simulink model "InnerOuter_Sim"  (Simulink 6.6)
settings: Solver=ode4  StartTime=0.0  StopTime=125  FixedStep=SampleT  RelTol=1e-3
InitFcn:
  | clc
  | innerOuterInit
undefined symbols (not defined in the file): A1, Apolar, apSampleTime, bankCommandLimit, baseHeight, baseTemp, CD0, chord, CL0, CLa, CLa_dot, Clb, ClDa, CLDe, CLDf, ClDr, clock, Clp, CLq, Clr, Cm0, Cma, CmDe, CmDf, Cmq, Cnb, CnDa, CnDr, Cnp, Cnr, compensatorOn, CYb, CYDr, da_failamp, da_failbias, da_failper, daL_fail, daLimit, daR_fail, deg, deLimit, derivativesConstant, dr_fail, dr_failamp, dr_failbias, dr_failper, drLimit, dtLimit, Earth, elarm, Euler_0, F, gaind, getWP, ISA_g, Ixx, Iyy, Izz, L1OF, L2_base ... (+28)
libraries: simulink x102, SLUGS_Library x23, aerolibconvert2 x15, dsPICdrivers x8, aerolibactuator x5, aerolibtransform2 x2, aerolibwind2 x2, dspmtrx3 x2, aerolibatmos2 x1, aerolibutil x1
(part 1 of 4)
CloseFcn:
  | rtwprivate ssgencode ModelCloseRequest AttitudeComplementary
settings Model: Creator=ASL_Lab  LastModifiedBy=Administrator
settings DebuggingCC: ConsistencyChecking=warning  AlgebraicLoopMsg=error  MultiTaskDSMMsg=warning  MultiTaskCondExecSysMsg=none  ModelReferenceExtraNoncontSigs=warning  StrictBusMsg=None
settings HardwareCC: TargetHWDeviceType=32-bit Generic
settings RTWCC: IncludeERTFirstTime=on

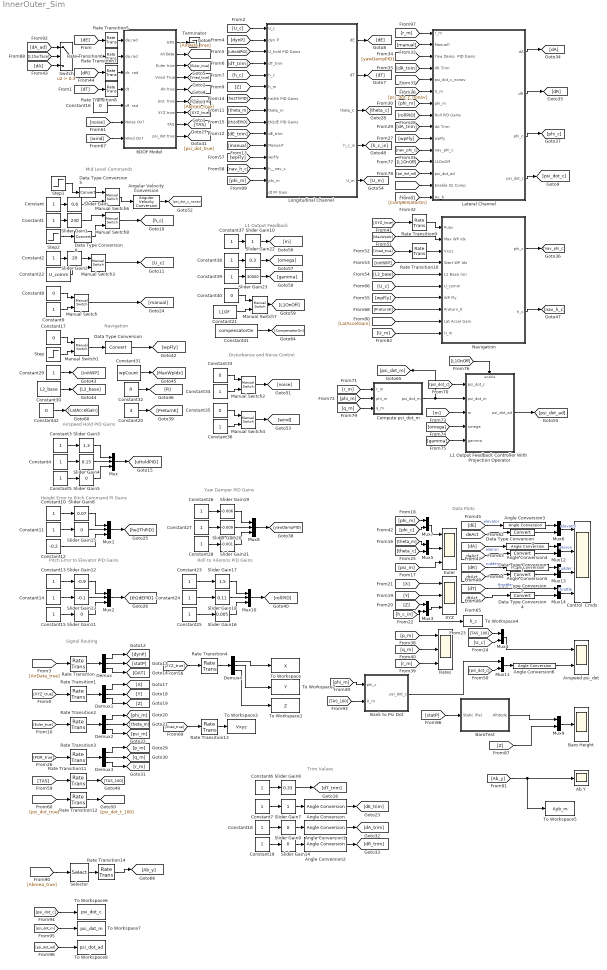
== system InnerOuter_Sim ==
  note: Mid Level Commands
  note: Trim Values
  note: Signal Routing
  note: Airspeed Hold PID Gains
  note: Height Error to Pitch Command PI Gains
  note: Pitch Error to Elevator PID Gains
  note: Data Plots
  note: Yaw Damper PID Gains
  note: Roll to Ailerons PID Gains
  note: Navigation
  note: Disturbance and Noise Control
  note: L1 Output Feedback
  6DOF Model : Subsystem
  Ab Y : Scope
      settings: TimeRange=140  YMin=-3  YMax=3  SaveName=ScopeData9
  Airspeed psi_dot : Scope  NumInputPorts=2
      settings: TimeRange=125  YMin=14.91~-37.5  YMax=15.05~5  SaveName=AirspeedPsiDot
  Angle Conversion : aerolibconvert2/Angle Conversion  SystemSampleTime=-1  IU=deg  OU=rad
  Angle Conversion1 : aerolibconvert2/Angle Conversion  SystemSampleTime=-1  IU=deg  OU=rad
  Angle Conversion2 : aerolibconvert2/Angle Conversion  SystemSampleTime=-1  IU=deg  OU=rad
  Angle Conversion{3..6} (4 alike) : aerolibconvert2/Angle Conversion  SystemSampleTime=-1  IU=rad  OU=deg
  Angular Velocity Conversion : aerolibconvert2/Angular Velocity Conversion  SystemSampleTime=-1  IU=deg/s  OU=rad/s
  Bank to Psi Dot : Subsystem  AncestorBlock=SLUGS_Library/Navigation/Bank to Psi Dot
  Baro Height : Scope
      settings: TimeRange=350  YMin=-1500  YMax=700  SaveName=AirspeedPsiDot1
  BaroTest : Subsystem
  Compute psi_dot_m : Subsystem
  Constant{,1..7,10..11,13..15,18..19,23..28,37..39} (24 alike) : Constant  OutDataTypeMode=single  SampleTime=apSampleTime
  Constant12 : Constant  Value=-0.2  OutDataTypeMode=single  SampleTime=apSampleTime
  Constant16 : Constant  Value=0
  Constant17 : Constant  Value=0  OutDataTypeMode=uint8  SampleTime=apSampleTime
  Constant20 : Constant  Value=4  SampleTime=apSampleTime
  Constant21 : Constant  Value=L1OF  SampleTime=apSampleTime
  Constant22 : Constant  Value=U_comm  SampleTime=apSampleTime
  Constant29 : Constant  OutDataTypeMode=uint8  SampleTime=apSampleTime
  Constant30 : Constant  Value=L2_base  OutDataTypeMode=single  SampleTime=apSampleTime
  Constant31 : Constant  Value=wpCount  SampleTime=apSampleTime
  Constant32 : Constant  Value=R  SampleTime=apSampleTime
  Constant33 : Constant  Value=0  SampleTime=SampleT
  Constant34 : Constant  SampleTime=SampleT
  Constant35 : Constant  Value=0  SampleTime=SampleT
  Constant36 : Constant  SampleTime=SampleT
  Constant40 : Constant  Value=0  OutDataTypeMode=uint8  SampleTime=apSampleTime
  Constant41 : Constant  Value=compensatorOn  SampleTime=apSampleTime
  Constant42 : Constant  Value=0  SampleTime=apSampleTime
  Constant8 : Constant  Value=0  OutDataTypeMode=uint8  SampleTime=apSampleTime
  Constant9 : Constant  OutDataTypeMode=uint8  SampleTime=apSampleTime
  Control  Cmds : Scope  NumInputPorts=4
      settings: TickLabels=on  TimeRange=100  YMin=-2~-10~-11~0.225  YMax=3.5~17.5~1~0.425  SaveName=ctrlCmds
  Data Type Conversion : DataTypeConversion  OutDataTypeMode=uint8
  Data Type Conversion{1..6} (6 alike) : DataTypeConversion  OutDataTypeMode=single
  Demux{,1..4} (5 alike) : Demux  Outputs=3
  Euler : Scope  NumInputPorts=3
      settings: TimeRange=100  YMin=-0.4~-0.02~0  YMax=1~0.06~7  SaveName=EulerData  DataFormat=Structure
  L1 Output Feedback Controller With  Projection Operator : Subsystem  TreatAsAtomicUnit=on
  Lateral Channel : Subsystem  TreatAsAtomicUnit=on
  Longitudinal Channel : Subsystem  TreatAsAtomicUnit=on
  Manual Switch{,2,4,6..8} (6 alike) : simulink/Signal Routing/Manual Switch  SystemSampleTime=-1  sw=1  action=0  varsize=off
  Manual Switch1 : simulink/Signal Routing/Manual Switch  SystemSampleTime=-1  sw=0  action=0  varsize=off
  Manual Switch3 : simulink/Signal Routing/Manual Switch  SystemSampleTime=-1  sw=0  action=0  varsize=off
  Mux{,1..2,8,10} (5 alike) : Mux  Inputs=3
  Mux{3..7,9,11..14} (10 alike) : Mux  Inputs=2
  Navigation : Subsystem  TreatAsAtomicUnit=on
  Rate Transition{,1..4,9..14} (11 alike) : RateTransition  OutPortSampleTime=apSampleTime
  Rate Transition{5..8} (4 alike) : RateTransition  OutPortSampleTime=SampleT
  Rates : Scope  NumInputPorts=3
      settings: TimeRange=300  YMin=-0.75~-1.5~-0.3  YMax=1~1.5~0.7  SaveName=ScopeData3
  Selector : Selector  IndexOptions=Index vector (dialog)  Indices=[2]  OutputSizes=1  InputPortWidth=3
  Slider Gain : simulink/Math Operations/Slider Gain  SystemSampleTime=-1  low=-18  gain=0.6  high=18
  Slider Gain1 : simulink/Math Operations/Slider Gain  SystemSampleTime=-1  low=0  gain=230  high=800
  Slider Gain10 : simulink/Math Operations/Slider Gain  SystemSampleTime=-1  low=0  gain=1  high=10
  Slider Gain11 : simulink/Math Operations/Slider Gain  SystemSampleTime=-1  low=-0.1  gain=0  high=0
  Slider Gain12 : simulink/Math Operations/Slider Gain  SystemSampleTime=-1  low=-2  gain=-0.9  high=0.3
  Slider Gain13 : simulink/Math Operations/Slider Gain  SystemSampleTime=-1  low=-0.1  gain=-0.1  high=0
  Slider Gain14 : simulink/Math Operations/Slider Gain  SystemSampleTime=-1  low=-10  gain=0  high=10
  Slider Gain15 : simulink/Math Operations/Slider Gain  SystemSampleTime=-1  low=-20  gain=0  high=20
  Slider Gain16 : simulink/Math Operations/Slider Gain  SystemSampleTime=-1  low=-0.1  gain=0.005  high=0.1
  Slider Gain17 : simulink/Math Operations/Slider Gain  SystemSampleTime=-1  low=-0.1  gain=1.5  high=5
  Slider Gain18 : simulink/Math Operations/Slider Gain  SystemSampleTime=-1  low=0  gain=0.11  high=2
  Slider Gain19 : simulink/Math Operations/Slider Gain  SystemSampleTime=-1  low=-20  gain=-0.006  high=20
  Slider Gain2 : simulink/Math Operations/Slider Gain  SystemSampleTime=-1  low=1  gain=20  high=55
  Slider Gain20 : simulink/Math Operations/Slider Gain  SystemSampleTime=-1  low=-20  gain=-0.009  high=20
  Slider Gain21 : simulink/Math Operations/Slider Gain  SystemSampleTime=-1  low=-20  gain=-0.001  high=20
  Slider Gain22 : simulink/Math Operations/Slider Gain  SystemSampleTime=-1  low=0  gain=0.3  high=5
  Slider Gain23 : simulink/Math Operations/Slider Gain  SystemSampleTime=-1  low=-50000  gain=30000  high=50000
  Slider Gain3 : simulink/Math Operations/Slider Gain  SystemSampleTime=-1  low=0  gain=1.3  high=4.5
  Slider Gain4 : simulink/Math Operations/Slider Gain  SystemSampleTime=-1  low=-20  gain=0.15  high=20
  Slider Gain5 : simulink/Math Operations/Slider Gain  SystemSampleTime=-1  low=-20  gain=0  high=20
  Slider Gain6 : simulink/Math Operations/Slider Gain  SystemSampleTime=-1  low=0.1  gain=0.33  high=1
  Slider Gain7 : simulink/Math Operations/Slider Gain  SystemSampleTime=-1  low=-10  gain=1  high=10
  Slider Gain8 : simulink/Math Operations/Slider Gain  SystemSampleTime=-1  low=-20  gain=0.07  high=20
  Slider Gain9 : simulink/Math Operations/Slider Gain  SystemSampleTime=-1  low=-10  gain=0  high=10
  Step : Step  Time=2  SampleTime=0.01
  Step1 : Step  Time=10  After=5  SampleTime=0.01
  Step2 : Step  Time=10  Before=Pos_0(3)  After=500  SampleTime=0.01
  Switch : Switch  Criteria=u2 > Threshold  Threshold=0.3  SampleTime=apSampleTime  InputSameDT=on
  Terminator : Terminator
  To Workspace : ToWorkspace  VariableName=X  SampleTime=-1  SaveFormat=Array
  To Workspace1 : ToWorkspace  VariableName=Z  SampleTime=-1  SaveFormat=Array
  To Workspace2 : ToWorkspace  VariableName=Y  SampleTime=-1  SaveFormat=Array
  To Workspace3 : ToWorkspace  VariableName=Vxyz  SampleTime=-1  SaveFormat=Array
  To Workspace4 : ToWorkspace  VariableName=h_c  SampleTime=-1  SaveFormat=Array
  To Workspace5 : ToWorkspace  VariableName=Ayb_m  SampleTime=.01  SaveFormat=Array
  To Workspace6 : ToWorkspace  VariableName=psi_dot_c  SampleTime=.01  SaveFormat=Array
  To Workspace7 : ToWorkspace  VariableName=psi_dot_m  SampleTime=.01  SaveFormat=Array
  To Workspace8 : ToWorkspace  VariableName=psi_dot_ad  SampleTime=.01  SaveFormat=Array
  XYZ : Scope  NumInputPorts=3
      settings: TimeRange=125  YMin=-250~-200~180  YMax=100~200~230
  wires:
  6DOF Model/7(XYZ true) -> [XYZ_true]
  6DOF Model/4(Vned True) -> [Vned_true]
  6DOF Model/5(Ab true) -> [Abmea_true]
  6DOF Model/6("pqr, true") -> [PQR_true]
  6DOF Model/3(Euler true) -> [Euler_true]
  6DOF Model/2(AirData) -> [AirData_true]
  Longitudinal Channel/1(dE) -> [dE]
  Longitudinal Channel/2(dT) -> [dT]
  Constant/1 -> Slider Gain/1
  Constant1/1 -> Slider Gain1/1
  Constant2/1 -> Slider Gain2/1
  Angular Velocity Conversion/1 -> [psi_dot_c_nonav]
  [U_c] -> Longitudinal Channel/1(U_c)
  [AirData_true] -> Rate Transition/1
  Demux/1 -> [dynP]
  Demux/2 -> [statP]
  Demux/3 -> [OAT]
  Constant3/1 -> Slider Gain3/1
  Constant4/1 -> Slider Gain4/1
  Constant5/1 -> Slider Gain5/1
  Slider Gain4/1 -> Mux/2
  Slider Gain3/1 -> Mux/1
  Slider Gain5/1 -> Mux/3
  Mux/1 -> [uHoldPID]
  [dynP] -> Longitudinal Channel/2(dyn P)
  [uHoldPID] -> Longitudinal Channel/3(U_hold PID Gains)
  Constant6/1 -> Slider Gain6/1
  Slider Gain6/1 -> [dT_trim]
  [dT_trim] -> Longitudinal Channel/4(dT_trim)
  [h_c] -> Longitudinal Channel/5(h_c)
  [XYZ_true] -> Rate Transition1/1
  Demux1/1 -> [X]
  Demux1/2 -> [Y]
  Demux1/3 -> [Z]
  [Z] -> Longitudinal Channel/6(h_m)
  [Euler_true] -> Rate Transition2/1
  Demux2/1 -> [phi_m]
  Demux2/2 -> [theta_m]
  Demux2/3 -> [psi_m]
  [theta_m] -> Longitudinal Channel/8(theta_m)
  Constant7/1 -> Slider Gain7/1
  Slider Gain7/1 -> Angle Conversion/1
  Angle Conversion/1 -> [dE_trim]
  [dE_trim] -> Longitudinal Channel/10(dE_trim)
  Constant8/1 -> Manual Switch/1
  Constant9/1 -> Manual Switch/2
  Manual Switch/1 -> [manual]
  [manual] -> Longitudinal Channel/11(Manual?)
  Constant10/1 -> Slider Gain8/1
  Constant11/1 -> Slider Gain15/1
  Constant12/1 -> Mux1/3
  Slider Gain8/1 -> Mux1/1
  Mux1/1 -> [he2ThPID]
  Constant13/1 -> Slider Gain12/1
  Constant14/1 -> Slider Gain13/1
  Constant15/1 -> Slider Gain11/1
  Slider Gain13/1 -> Mux2/2
  Slider Gain12/1 -> Mux2/1
  Slider Gain11/1 -> Mux2/3
  Mux2/1 -> [th2dEPID]
  [he2ThPID] -> Longitudinal Channel/7(he2th PID Gains)
  [th2dEPID] -> Longitudinal Channel/9(th2dE PID Gains)
  Mux5/1 -> Euler/2
  [psi_m] -> Euler/3
  [X] -> XYZ/1
  [Y] -> XYZ/2
  Mux3/1 -> XYZ/3
  [Z] -> Mux3/1
  [h_c_in] -> Mux3/2, To Workspace4/1
  [dT] -> Rate Transition8/1
  [dE] -> Rate Transition5/1
  Mux4/1 -> Airspeed psi_dot/1
  6DOF Model/8(TAS) -> [TAS]
  [TAS_100] -> Mux4/1
  [U_c] -> Mux4/2
  [theta_c] -> Mux5/2
  Longitudinal Channel/3(theta_C) -> [theta_c]
  [PQR_true] -> Rate Transition3/1
  Demux3/1 -> [p_m]
  Demux3/2 -> [q_m]
  Demux3/3 -> [r_m]
  Constant18/1 -> Slider Gain9/1
  Slider Gain9/1 -> Angle Conversion1/1
  Angle Conversion1/1 -> [dA_trim]
  Constant19/1 -> Slider Gain14/1
  Slider Gain14/1 -> Angle Conversion2/1
  Angle Conversion2/1 -> [dR_trim]
  [Ab_y] -> Lateral Channel/15(Ay_b)
  [manual] -> Lateral Channel/2(Manual?)
  [yawDampPID] -> Lateral Channel/3(Yaw Damp  PID Gains)
  [dR_trim] -> Lateral Channel/4(dR Trim)
  [psi_dot_c_nonav] -> Lateral Channel/5(psi_dot_c_nonav)
  [U_m] -> Lateral Channel/6(U_m)
  [phi_m] -> Lateral Channel/7(phi_m)
  [rollPID] -> Lateral Channel/8(Roll PID Gains)
  [dA_trim] -> Lateral Channel/9(dA Trim)
  [r_m] -> Rates/3
  Lateral Channel/3(phi_c) -> [phi_c]
  [q_m] -> Rates/2
  [phi_m] -> Mux7/1
  [phi_c] -> Mux7/2
  Mux7/1 -> Euler/1
  Constant26/1 -> Slider Gain19/1
  Constant27/1 -> Slider Gain20/1
  Constant28/1 -> Slider Gain21/1
  Slider Gain20/1 -> Mux8/2
  Slider Gain19/1 -> Mux8/1
  Slider Gain21/1 -> Mux8/3
  Mux8/1 -> [yawDampPID]
  Constant23/1 -> Slider Gain17/1
  Constant24/1 -> Slider Gain18/1
  Constant25/1 -> Slider Gain16/1
  Slider Gain18/1 -> Mux10/2
  Slider Gain17/1 -> Mux10/1
  Slider Gain16/1 -> Mux10/3
  Mux10/1 -> [rollPID]
  Switch/1 -> Rate Transition6/1
  [dR] -> Rate Transition7/1
  Constant16/1 -> 6DOF Model/5("df, rad")
  Slider Gain15/1 -> Mux1/2
  Mux6/1 -> Control  Cmds/1  "elevator"
  Mux12/1 -> Control  Cmds/2  "aileron"
  [theta_m] -> Mux5/1
  6DOF Model/9(psi_dot true) -> [psi_dot_true]
  Bank to Psi Dot/1(psi_dot_c) -> Mux11/1
  [psi_dot_c] -> Mux11/2
  Mux11/1 -> Angle Conversion6/1
  [p_m] -> Rates/1
  Constant17/1 -> Manual Switch1/1
  Step/1 -> Manual Switch1/2
  Manual Switch1/1 -> Data Type Conversion/1
  Constant29/1 -> [initWP]
  [wpFly] -> Lateral Channel/10(wpFly)
  Navigation/1(phi_c) -> [nav_phi_c]
  [nav_phi_c] -> Lateral Channel/11(nav_phi_c)
  [XYZ_true] -> Rate Transition9/1
  Constant30/1 -> [L2_base]
  Constant31/1 -> [MaxWpIdx]
  [Vned_true] -> Rate Transition10/1
  [L2_base] -> Navigation/5(L2 Base (m))
  [XYZ_true] -> Rate Transition4/1
  Demux4/1 -> To Workspace/1
  Demux4/2 -> To Workspace2/1
  Demux4/3 -> To Workspace1/1
  Navigation/2(h_c) -> [nav_h_c]
  [wpFly] -> Longitudinal Channel/12(wpFly)
  [nav_h_c] -> Longitudinal Channel/13(h__nav_c)
  Longitudinal Channel/4(h_c_in) -> [h_c_in]
  Rate Transition/1 -> Demux/1
  Rate Transition1/1 -> Demux1/1
  Rate Transition2/1 -> Demux2/1
  Rate Transition3/1 -> Demux3/1
  Rate Transition4/1 -> Demux4/1
  Rate Transition9/1 -> Navigation/1(Puav)
  Rate Transition10/1 -> Navigation/3(Vxyz)
  [TAS] -> Rate Transition11/1
  Rate Transition11/1 -> [TAS_100]
  [psi_dot_true] -> Rate Transition12/1
  Rate Transition12/1 -> [psi_dot_t_100]
  Constant33/1 -> Manual Switch2/1
  Constant34/1 -> Manual Switch2/2
  Manual Switch2/1 -> [noise]
  [noise] -> 6DOF Model/6(Noise On?)
  Constant32/1 -> [R]
  [U_c] -> Navigation/6(U_comm)
  6DOF Model/1(GPS) -> Terminator/1
  [wpFly] -> Navigation/7(WP Fly)
  Slider Gain2/1 -> Manual Switch3/1
  Manual Switch3/1 -> [U_c]
  Constant22/1 -> Manual Switch3/2
  [dE] -> Angle Conversion3/1  "elevator"
  [deAct] -> Data Type Conversion3/1
  [dA] -> Angle Conversion4/1  "aileron"
  [daAct] -> Data Type Conversion1/1
  Mux13/1 -> Control  Cmds/3  "rudder"
  [dR] -> Angle Conversion5/1  "rudder"
  [drAct] -> Data Type Conversion2/1
  Mux14/1 -> Control  Cmds/4  "throttle"
  [dT] -> Mux14/1  "throttle"
  [dtAct] -> Data Type Conversion4/1
  Lateral Channel/4("psi_dot_c ") -> [psi_dot_c]
  Constant35/1 -> Manual Switch4/1
  Constant36/1 -> Manual Switch4/2
  Manual Switch4/1 -> [wind]
  [wind] -> 6DOF Model/7(Wind On?)
  Longitudinal Channel/5(U_m) -> [U_m]
  Data Type Conversion/1 -> [wpFly]
  Lateral Channel/1(dA) -> [dA]
  Lateral Channel/2(dR) -> [dR]
  Data Type Conversion3/1 -> Mux6/2
  Data Type Conversion1/1 -> Mux12/2
  Data Type Conversion2/1 -> Mux13/2
  Data Type Conversion4/1 -> Mux14/2
  Rate Transition5/1 -> 6DOF Model/1(de,rad)
  Rate Transition8/1 -> 6DOF Model/4(dt)
  Rate Transition6/1 -> 6DOF Model/2(da,rad)
  Rate Transition7/1 -> 6DOF Model/3("dr, rad")
  Rate Transition13/1 -> To Workspace3/1
  [Vned_true] -> Rate Transition13/1
  Manual Switch6/1 -> Angular Velocity Conversion/1
  Slider Gain/1 -> Manual Switch6/2
  Step1/1 -> Data Type Conversion5/1
  Data Type Conversion5/1 -> Manual Switch6/1
  [psi_dot_c] -> L1 Output Feedback Controller With  Projection Operator/1(psi_dot_c)
  L1 Output Feedback Controller With  Projection Operator/1(psi_dot_ad) -> [psi_dot_ad]
  [phi_m] -> Compute psi_dot_m/2(phi_m)
  [r_m] -> Compute psi_dot_m/1(r_m)
  Constant37/1 -> Slider Gain10/1
  Slider Gain10/1 -> [m]
  Constant38/1 -> Slider Gain22/1
  Slider Gain22/1 -> [omega]
  Constant39/1 -> Slider Gain23/1
  Slider Gain23/1 -> [gamma]
  [m] -> L1 Output Feedback Controller With  Projection Operator/3(m)
  [omega] -> L1 Output Feedback Controller With  Projection Operator/4(omega)
  [gamma] -> L1 Output Feedback Controller With  Projection Operator/5(gamma)
  Constant40/1 -> Manual Switch7/1
  Constant21/1 -> Manual Switch7/2
  Manual Switch7/1 -> [L1OnOff]
  [L1OnOff] -> Lateral Channel/12(L1OnOff)
  [psi_dot_ad] -> Lateral Channel/13(psi_dot_ad)
  [L1OnOff] -> L1 Output Feedback Controller With  Projection Operator/Enable
  [q_m] -> Compute psi_dot_m/3(q_m)
  Compute psi_dot_m/1(psi_dot_m) -> L1 Output Feedback Controller With  Projection Operator/2(psi_dot_m), [psi_dot_m]
  Angle Conversion3/1 -> Mux6/1
  Angle Conversion4/1 -> Mux12/1
  Angle Conversion5/1 -> Mux13/1
  [dA] -> Switch/3
  [dA_ad] -> Switch/1
  [L1Surface] -> Switch/2
  Constant41/1 -> [CompensatorOn]
  [CompensatorOn] -> Lateral Channel/14(Enable SS Comp)
  Manual Switch8/1 -> [h_c]
  Step2/1 -> Data Type Conversion6/1
  Slider Gain1/1 -> Manual Switch8/1
  Data Type Conversion6/1 -> Manual Switch8/2
  [statP] -> BaroTest/1(Static (Pa))
  Mux9/1 -> Baro Height/1
  [Z] -> Mux9/2
  BaroTest/1(Altitude) -> Mux9/1
  [phi_m] -> Longitudinal Channel/14(phi_m)
  Selector/1 -> Rate Transition14/1
  [Abmea_true] -> Selector/1
  Rate Transition14/1 -> [Ab_y]
  [Ab_y] -> Ab Y/1, To Workspace5/1
  Angle Conversion6/1 -> Airspeed psi_dot/2
  [phi_m] -> Bank to Psi Dot/1(phi_c)
  [TAS_100] -> Bank to Psi Dot/2(U_m)
  [psi_dot_c] -> To Workspace6/1
  [psi_dot_m] -> To Workspace7/1
  [psi_dot_ad] -> To Workspace8/1
  [r_m] -> Lateral Channel/1(r_m)
  [MaxWpIdx] -> Navigation/2(Max WP Idx)
  [initWP] -> Navigation/4(Start WP Idx)
  [PreturnK] -> Navigation/8(Preturn_K)
  Constant20/1 -> [PreturnK]
  Constant42/1 -> [LatAccelGain]
  [LatAccelGain] -> Navigation/9(Lat Accel Gain)
  [U_m] -> Navigation/10(U_m)

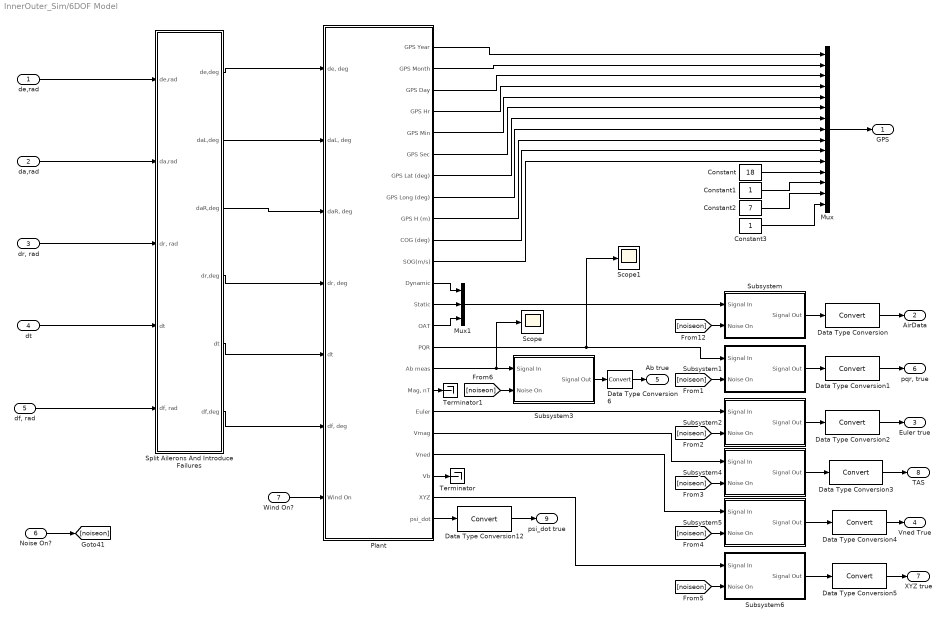
== system InnerOuter_Sim/6DOF Model ==
  de,rad : Inport
  da,rad : Inport  Port=2
  "dr, rad" : Inport  Port=3
  dt : Inport  Port=4
  "df, rad" : Inport  Port=5
  Noise On? : Inport  Port=6
  Wind On? : Inport  Port=7
  Constant : Constant  Value=18  SampleTime=SampleT
  Constant1 : Constant  SampleTime=SampleT
  Constant2 : Constant  Value=7  SampleTime=SampleT
  Constant3 : Constant  SampleTime=SampleT
  Data Type Conversion{,1..6,12} (8 alike) : DataTypeConversion  OutDataTypeMode=single
  Mux : Mux  Inputs=15
  Mux1 : Mux  Inputs=3
  Plant : Subsystem
  Scope : Scope
      settings: YMin=-13  YMax=1  SaveName=ScopeData5
  Scope1 : Scope
      settings: YMin=-0.05  YMax=0.04  SaveName=ScopeData6
  Split Ailerons And Introduce Failures : Subsystem
  Subsystem : Subsystem  mask{nv=[0.01 0.01 0.1], st=SampleT, ns=[132 564 987]}
      mask prompts: nv "Noise Variance"; st "Sample Time"; ns "Noise Seed"
  Subsystem1 : Subsystem  mask{nv=[0.001 0.001 0.001], st=SampleT, ns=[132 564 987]}
      mask prompts: nv "Noise Variance"; st "Sample Time"; ns "Noise Seed"
  Subsystem2 : Subsystem  mask{nv=[0.0001 0.00003 0.0001], st=SampleT, ns=[132 564 987]}
      mask prompts: nv "Noise Variance"; st "Sample Time"; ns "Noise Seed"
  Subsystem3 : Subsystem  mask{nv=[0.1 0.1 0.1], st=SampleT, ns=[132 564 987]}
      mask prompts: nv "Noise Variance"; st "Sample Time"; ns "Noise Seed"
  Subsystem4 : Subsystem  mask{nv=[0.01], st=SampleT, ns=[321564]}
      mask prompts: nv "Noise Variance"; st "Sample Time"; ns "Noise Seed"
  Subsystem5 : Subsystem  mask{nv=[0.01 0.01 0.01], st=SampleT, ns=[321564 6546 98798]}
      mask prompts: nv "Noise Variance"; st "Sample Time"; ns "Noise Seed"
  Subsystem6 : Subsystem  mask{nv=[0.05 0.05 0.07], st=SampleT, ns=[321564]}
      mask prompts: nv "Noise Variance"; st "Sample Time"; ns "Noise Seed"
  Terminator : Terminator
  Terminator1 : Terminator
  GPS : Outport
  AirData : Outport  Port=2
  Euler true : Outport  Port=3
  Vned True : Outport  Port=4
  Ab true : Outport  Port=5
  "pqr, true" : Outport  Port=6
  XYZ true : Outport  Port=7
  TAS : Outport  Port=8
  psi_dot true : Outport  Port=9
  wires:
  Mux/1 -> GPS/1
  Plant/1(GPS Year) -> Mux/1
  Plant/2(GPS Month) -> Mux/2
  Plant/3(GPS Day) -> Mux/3
  Plant/4(GPS Hr) -> Mux/4
  Plant/5(GPS Min) -> Mux/5
  Plant/6(GPS Sec) -> Mux/6
  Plant/7(GPS Lat (deg)) -> Mux/7
  Plant/8(GPS Long (deg)) -> Mux/8
  Plant/9(GPS H (m)) -> Mux/9
  Plant/10(COG (deg)) -> Mux/10
  Plant/11(SOG(m/s)) -> Mux/11
  Plant/12(Dynamic) -> Mux1/1
  Plant/13(Static) -> Mux1/2
  Plant/14(OAT) -> Mux1/3
  Mux1/1 -> Subsystem/1(Signal In)
  Constant/1 -> Mux/12
  Constant1/1 -> Mux/13
  Constant2/1 -> Mux/14
  Constant3/1 -> Mux/15
  Plant/23(psi_dot) -> Data Type Conversion12/1
  Noise On?/1 -> [noiseon]
  Subsystem/1(Signal Out) -> Data Type Conversion/1
  [noiseon] -> Subsystem/2(Noise On)
  [noiseon] -> Subsystem1/2(Noise On)
  [noiseon] -> Subsystem2/2(Noise On)
  [noiseon] -> Subsystem4/2(Noise On)
  [noiseon] -> Subsystem5/2(Noise On)
  [noiseon] -> Subsystem6/2(Noise On)
  [noiseon] -> Subsystem3/2(Noise On)
  Subsystem1/1(Signal Out) -> Data Type Conversion1/1
  Plant/15(PQR) -> Subsystem1/1(Signal In), Scope1/1
  Subsystem2/1(Signal Out) -> Data Type Conversion2/1
  Plant/18(Euler) -> Subsystem2/1(Signal In)
  Subsystem3/1(Signal Out) -> Data Type Conversion6/1
  Plant/16(Ab meas) -> Subsystem3/1(Signal In), Scope/1
  Subsystem4/1(Signal Out) -> Data Type Conversion3/1
  Plant/19(Vmag) -> Subsystem4/1(Signal In)
  Subsystem5/1(Signal Out) -> Data Type Conversion4/1
  Plant/20(Vned) -> Subsystem5/1(Signal In)
  Subsystem6/1(Signal Out) -> Data Type Conversion5/1
  Plant/22(XYZ) -> Subsystem6/1(Signal In)
  Plant/21(Vb) -> Terminator/1
  Plant/17("Mag, nT") -> Terminator1/1
  Split Ailerons And Introduce Failures/1(de,deg) -> Plant/1("de, deg")
  Split Ailerons And Introduce Failures/6(df,deg) -> Plant/6("df, deg")
  Split Ailerons And Introduce Failures/4(dr,deg) -> Plant/4("dr, deg")
  Split Ailerons And Introduce Failures/2(daL,deg) -> Plant/2("daL, deg")
  Wind On?/1 -> Plant/7(Wind On)
  Data Type Conversion/1 -> AirData/1
  Data Type Conversion1/1 -> "pqr, true"/1
  Data Type Conversion2/1 -> Euler true/1
  Data Type Conversion3/1 -> TAS/1
  Data Type Conversion4/1 -> Vned True/1
  Data Type Conversion5/1 -> XYZ true/1
  Data Type Conversion6/1 -> Ab true/1
  Data Type Conversion12/1 -> psi_dot true/1
  de,rad/1 -> Split Ailerons And Introduce Failures/1(de,rad)
  da,rad/1 -> Split Ailerons And Introduce Failures/2(da,rad)
  "dr, rad"/1 -> Split Ailerons And Introduce Failures/3("dr, rad")
  dt/1 -> Split Ailerons And Introduce Failures/4(dt)
  Split Ailerons And Introduce Failures/5("dt ") -> Plant/5(dt)
  "df, rad"/1 -> Split Ailerons And Introduce Failures/5("df, rad")
  Split Ailerons And Introduce Failures/3(daR,deg) -> Plant/3("daR, deg")

== system InnerOuter_Sim/Bank to Psi Dot ==
  phi_c : Inport
  U_m : Inport  Port=2
  Constant1 : Constant  Value=9.80665  OutDataTypeMode=single
  Divide : Product  Inputs=/*  OutDataTypeMode=single  OutScaling=2^-10  SampleTime=apSampleTime
  Divide1 : Product  OutDataTypeMode=single  OutScaling=2^-10  SampleTime=apSampleTime
  Subsystem8 : SLUGS_Library/Subsystem8  SystemSampleTime=-1
  negprotect : Stateflow chart
  psi_dot_c : Outport
  wires:
  negprotect/1(zpVal) -> Divide/1
  Divide/1 -> Divide1/2
  phi_c/1 -> Subsystem8/1
  Subsystem8/1 -> Divide1/1
  Divide1/1 -> psi_dot_c/1
  Constant1/1 -> Divide/2
  U_m/1 -> negprotect/1(val)

== system InnerOuter_Sim/BaroTest ==
  Static (Pa) : Inport  Orientation=up
  Compute Barometric Height : Subsystem  mask{baseTemp=baseTemp, LapseRate=lapseRate}
      mask prompts: baseTemp "Base Station Temperature (K)"; LapseRate "Lapse Rate (C/ft)"
      mask help:
      | Produces Altitude in meters from Barometric Pressure in Pascals. Altitude is valid from MSL to 6000 ft.
      |
      | The method implemented here was developed by Ren Curry
  Constant1 : Constant  Value=baseHeight  OutDataTypeMode=single
  Enables/Disables the Computation of  initial Baro Bias : Stateflow chart
  Initial Baro Bias : Subsystem  TreatAsAtomicUnit=on
  Sum1 : Sum  Inputs=++|  OutDataTypeMode=single
  Zero Out Height : Subsystem  TreatAsAtomicUnit=on
  Altitude : Outport
  wires:
  Compute Barometric Height/1("Altitude, m") -> Zero Out Height/2(Computed Height), Sum1/2
  Static (Pa)/1 -> Initial Baro Bias/1(Baro (Pa)), Compute Barometric Height/3(Baro (Pa))
  Enables/Disables the Computation of  initial Baro Bias/1(tOut) -> Initial Baro Bias/Enable, Zero Out Height/Enable
  Constant1/1 -> Compute Barometric Height/1(Base Height (m)), Zero Out Height/1(Base Height)
  Initial Baro Bias/1(Baro (Gnd)) -> Compute Barometric Height/2(Base Pressure (Pa))
  Zero Out Height/1(Height Offset) -> Sum1/1
  Sum1/1 -> Altitude/1

== system InnerOuter_Sim/Compute psi_dot_m ==
  r_m : Inport
  phi_m : Inport  Port=2
  q_m : Inport  Port=3
  Product : Product  SampleTime=apSampleTime  RndMeth=Zero
  Product1 : Product  SampleTime=apSampleTime  RndMeth=Zero
  Subsystem5 : Subsystem  AncestorBlock=SLUGS_Library/Subsystem5
  Subsystem7 : SLUGS_Library/Subsystem7  SystemSampleTime=-1
  Subtract : Sum  Inputs=2  OutScaling=2^-10
  psi_dot_m : Outport
  wires:
  Subsystem5/1(cos(u)) -> Product/2
  Subsystem7/1 -> Product1/2
  Product/1 -> Subtract/1
  Product1/1 -> Subtract/2
  r_m/1 -> Product/1
  phi_m/1 -> Subsystem5/1(u), Subsystem7/1
  Subtract/1 -> psi_dot_m/1
  q_m/1 -> Product1/1

== system InnerOuter_Sim/L1 Output Feedback Controller With  Projection Operator ==
  psi_dot_c : Inport
  psi_dot_m : Inport  Port=2
  m : Inport  Port=3
  omega : Inport  Port=4
  gamma : Inport  Port=5
  Enable : EnablePort  ShowOutputPort=on
  Constant : Constant  Value=2  OutDataTypeMode=single
  Constant1 : Constant  OutDataTypeMode=single
  Control  Law : Subsystem
      mask Display:
      | droots([],'-a','a')
      | port_label('input',1,'a')
      | port_label('input',2,'u')
      | port_label('output',1,'y')
  Gain : Gain  Gain=-1
  Integer Delay : simulink/Discrete/Integer Delay  vinit=0.0  samptime=apSampleTime  NumDelays=1
  Integer Delay1 : simulink/Discrete/Integer Delay  Orientation=left  vinit=0.0  samptime=-1  NumDelays=1
  Logical Operator : Logic  Operator=NOT  AllPortsSameDT=off  OutDataTypeMode=Specify via dialog
  Projection : Product  SampleTime=apSampleTime  RndMeth=Zero
  Projection Operator : Subsystem
  Psi Dot  Limit : Saturate  UpperLimit=1  LowerLimit=-1  SampleTime=apSampleTime
  State Predictor : Subsystem
      mask Display:
      | droots([],'-a','a')
      | port_label('input',1,'a')
      | port_label('input',2,'u')
      | port_label('output',1,'y')
  Sum2 : Sum  Inputs=|++  SampleTime=apSampleTime
  Sum3 : Sum  Inputs=-+|  SampleTime=apSampleTime
  Sum4 : Sum  Inputs=+-|  SampleTime=apSampleTime
  Trapezoidal Integrator : Subsystem  AncestorBlock=SLUGS_Library/Control Blocks/PID Controller w//Anti-Windup/Trapezoidal Integrator  mask{T=apSampleTime, upperLimit=2, lowerLimit=-2}
      mask prompts: T "Sample Time"; upperLimit "Upper Saturation"; lowerLimit "Lower Saturation"
  psi_dot_ad : Outport
  wires:
  Integer Delay1/1 -> Projection Operator/3(Theta), Sum2/2
  Constant1/1 -> Projection Operator/2(Eps 0)
  Constant/1 -> Projection Operator/1(Theta Max)
  Projection Operator/1("Proj(the, y)") -> Projection/2  "G*Proj"
  Sum4/1 -> Psi Dot  Limit/1  "psi_ad"
  Control  Law/1(y) -> Sum4/2  "sigma_hat_fil"
  omega/1 -> Control  Law/1(a)
  psi_dot_c/1 -> Integer Delay/1  "psi_dot_c"
  Trapezoidal Integrator/1(Int(x)) -> Control  Law/2(u), Integer Delay1/1  "sigma_hat"
  Projection/1 -> Trapezoidal Integrator/1(x)
  gamma/1 -> Projection/1  "adaptation gain"
  Sum3/1 -> Gain/1  "psi_dot_tilde"
  psi_dot_m/1 -> Sum3/1  "psi_dot_m"
  Sum2/1 -> State Predictor/2(u)
  m/1 -> State Predictor/1(a)
  Gain/1 -> Projection Operator/4(y)
  State Predictor/1(y) -> Sum3/2
  Integer Delay/1 -> Sum4/1  "psi_dot_c"
  Psi Dot  Limit/1 -> psi_dot_ad/1, Sum2/1
  Logical Operator/1 -> Trapezoidal Integrator/2(Reset)
  Enable/1 -> Logical Operator/1

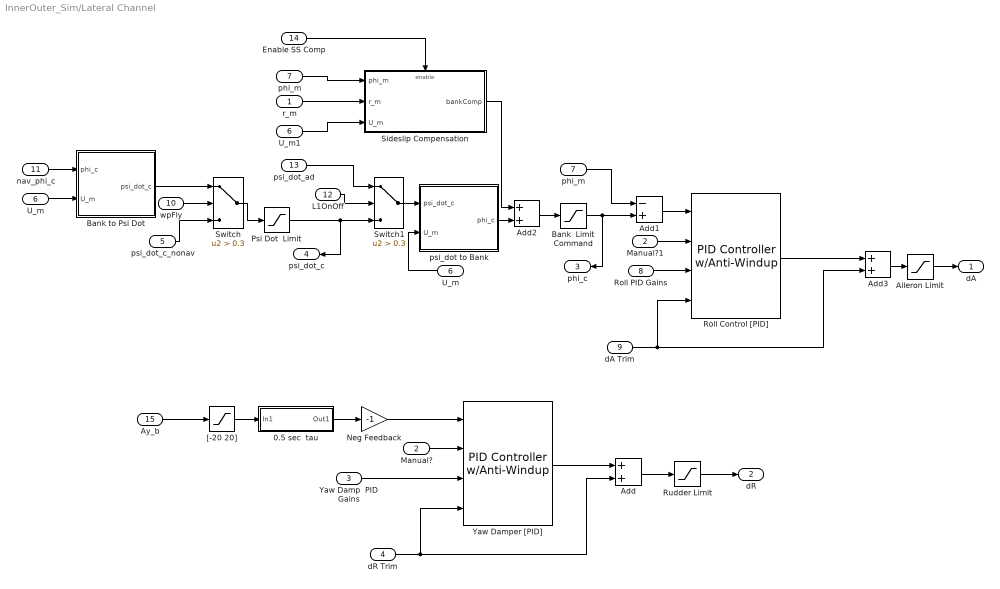
== system InnerOuter_Sim/Lateral Channel ==
  r_m : Inport
  Manual? : Inport  Port=2
  Yaw Damp  PID Gains : Inport  Port=3
  dR Trim : Inport  Port=4
  psi_dot_c_nonav : Inport  Port=5
  U_m : Inport  Port=6
  phi_m : Inport  Port=7
  Roll PID Gains : Inport  Port=8
  dA Trim : Inport  Port=9
  wpFly : Inport  Port=10  SampleTime=apSampleTime
  nav_phi_c : Inport  Port=11
  L1OnOff : Inport  Port=12  SampleTime=apSampleTime
  psi_dot_ad : Inport  Port=13  SampleTime=apSampleTime
  Enable SS Comp : Inport  Port=14
  Ay_b : Inport  Port=15
  0.5 sec  tau : Subsystem  mask(Tustin1stOrderLowpassAutoInitialCondition){f=0.3183, T=T}
      mask prompts: f "Lowpass Frequency"; T "Sample Time"
      mask help: Takes a 3db rolloff frequency (in Hz, NOT radians/s) and a sample time. Performs a symbolic Tustin conversion and implements in a discrete filter. The initial output of the filter is set by the first sample.
      mask Help: Enter the desired 3db rolloff frequency in Hz and the sample time. Initial conditions are sampled automatically.
      mask Display: fprintf('%.2f Hz lowpass',f)
  Add : Sum  OutDataTypeMode=single  OutScaling=2^-10
  Add1 : Sum  Inputs=-+  OutDataTypeMode=single  OutScaling=2^-10
  Add2 : Sum  OutDataTypeMode=single  OutScaling=2^-10
  Add3 : Sum  OutDataTypeMode=single  OutScaling=2^-10
  Aileron Limit : Saturate  UpperLimit=daLimit  LowerLimit=-daLimit  SampleTime=apSampleTime
  Bank  Limit Command : Saturate  UpperLimit=bankCommandLimit  LowerLimit=-bankCommandLimit  SampleTime=apSampleTime
  Bank to Psi Dot : Subsystem  AncestorBlock=SLUGS_Library/Navigation/Bank to Psi Dot
  Manual?1 : InportShadow  Port=2  LatchByCopyingInsideSignal=off
  Neg Feedback : Gain  Gain=-1  OutDataTypeMode=Specify via dialog  OutDataType=float('double')
  Psi Dot  Limit : Saturate  UpperLimit=1  LowerLimit=-1  SampleTime=apSampleTime
  Roll Control [PID] : SLUGS_Library/Control Blocks/PID Controller w//Anti-Windup  SystemSampleTime=-1  Tsample=apSampleTime  Ndelay=derivativesConstant  upperSaturationLimit=daLimit  lowerSaturationLimit=-daLimit
  Rudder Limit : Saturate  UpperLimit=drLimit  LowerLimit=-drLimit  SampleTime=apSampleTime
  Sideslip Compensation : Subsystem
  Switch : Switch  Criteria=u2 > Threshold  Threshold=0.3  SampleTime=apSampleTime
  Switch1 : Switch  Criteria=u2 > Threshold  Threshold=0.3  SampleTime=apSampleTime
  "U_m " : InportShadow  Orientation=left  Port=6  LatchByCopyingInsideSignal=off
  U_m1 : InportShadow  Port=6  LatchByCopyingInsideSignal=off
  Yaw Damper [PID] : SLUGS_Library/Control Blocks/PID Controller w//Anti-Windup  SystemSampleTime=-1  Tsample=apSampleTime  Ndelay=derivativesConstant  upperSaturationLimit=drLimit  lowerSaturationLimit=-drLimit
  "[-20 20]" : Saturate  UpperLimit=20  LowerLimit=-20
  "phi_m " : InportShadow  Port=7  LatchByCopyingInsideSignal=off
  psi_dot to Bank : Subsystem  AncestorBlock=SLUGS_Library/Navigation/psi_dot to Bank
  dA : Outport
  dR : Outport  Port=2
  phi_c : Outport  Orientation=left  Port=3
  "psi_dot_c " : Outport  Orientation=left  Port=4
  wires:
  Rudder Limit/1 -> dR/1
  Manual?/1 -> Yaw Damper [PID]/2
  Yaw Damp  PID Gains/1 -> Yaw Damper [PID]/3
  Add/1 -> Rudder Limit/1
  Yaw Damper [PID]/1 -> Add/1
  U_m/1 -> Bank to Psi Dot/2(U_m)
  Manual?1/1 -> Roll Control [PID]/2
  Roll PID Gains/1 -> Roll Control [PID]/3
  Add3/1 -> Aileron Limit/1
  Roll Control [PID]/1 -> Add3/1
  Aileron Limit/1 -> dA/1
  Add1/1 -> Roll Control [PID]/1
  phi_m/1 -> Add1/1
  Bank to Psi Dot/1(psi_dot_c) -> Switch/1
  wpFly/1 -> Switch/2
  Bank  Limit Command/1 -> Add1/2, phi_c/1
  nav_phi_c/1 -> Bank to Psi Dot/1(phi_c)
  Switch/1 -> Psi Dot  Limit/1
  "U_m "/1 -> psi_dot to Bank/2(U_m)
  psi_dot_c_nonav/1 -> Switch/3
  Switch1/1 -> psi_dot to Bank/1(psi_dot_c)
  L1OnOff/1 -> Switch1/2
  psi_dot_ad/1 -> Switch1/1
  "phi_m "/1 -> Sideslip Compensation/1(phi_m)
  r_m/1 -> Sideslip Compensation/2(r_m)
  U_m1/1 -> Sideslip Compensation/3(U_m)
  Add2/1 -> Bank  Limit Command/1
  psi_dot to Bank/1(phi_c) -> Add2/2
  Sideslip Compensation/1(bankComp) -> Add2/1
  Enable SS Comp/1 -> Sideslip Compensation/Enable
  Ay_b/1 -> "[-20 20]"/1
  Neg Feedback/1 -> Yaw Damper [PID]/1
  Psi Dot  Limit/1 -> Switch1/3, "psi_dot_c "/1
  dA Trim/1 -> Roll Control [PID]/4, Add3/2
  "[-20 20]"/1 -> 0.5 sec  tau/1(In1)
  0.5 sec  tau/1(Out1) -> Neg Feedback/1
  dR Trim/1 -> Yaw Damper [PID]/4, Add/2

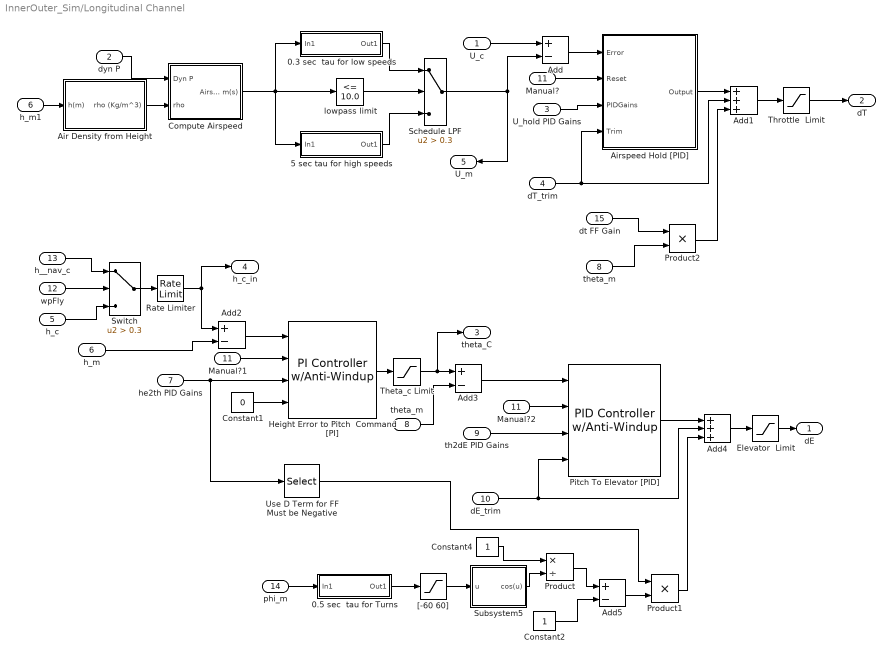
== system InnerOuter_Sim/Longitudinal Channel ==
  U_c : Inport
  dyn P : Inport  Port=2
  U_hold PID Gains : Inport  Port=3
  dT_trim : Inport  Port=4
  h_c : Inport  Port=5
  h_m : Inport  Port=6
  he2th PID Gains : Inport  Port=7
  theta_m : Inport  Port=8
  th2dE PID Gains : Inport  Port=9
  dE_trim : Inport  Port=10
  Manual? : Inport  Port=11
  wpFly : Inport  Port=12  SampleTime=apSampleTime
  h__nav_c : Inport  Port=13
  phi_m : Inport  Port=14
  dt FF Gain : Inport  Port=15
  0.3 sec  tau for low speeds : Subsystem  mask(Tustin1stOrderLowpassAutoInitialCondition){f=10, T=T}
      mask prompts: f "Lowpass Frequency"; T "Sample Time"
      mask help: Takes a 3db rolloff frequency (in Hz, NOT radians/s) and a sample time. Performs a symbolic Tustin conversion and implements in a discrete filter. The initial output of the filter is set by the first sample.
      mask Help: Enter the desired 3db rolloff frequency in Hz and the sample time. Initial conditions are sampled automatically.
      mask Display: fprintf('%.2f Hz lowpass',f)
  0.5 sec  tau for Turns : Subsystem  mask(Tustin1stOrderLowpassAutoInitialCondition){f=0.32, T=T}
      mask prompts: f "Lowpass Frequency"; T "Sample Time"
      mask help: Takes a 3db rolloff frequency (in Hz, NOT radians/s) and a sample time. Performs a symbolic Tustin conversion and implements in a discrete filter. The initial output of the filter is set by the first sample.
      mask Help: Enter the desired 3db rolloff frequency in Hz and the sample time. Initial conditions are sampled automatically.
      mask Display: fprintf('%.2f Hz lowpass',f)
  5 sec tau for high speeds : Subsystem  mask(Tustin1stOrderLowpassAutoInitialCondition){f=100, T=T}
      mask prompts: f "Lowpass Frequency"; T "Sample Time"
      mask help: Takes a 3db rolloff frequency (in Hz, NOT radians/s) and a sample time. Performs a symbolic Tustin conversion and implements in a discrete filter. The initial output of the filter is set by the first sample.
      mask Help: Enter the desired 3db rolloff frequency in Hz and the sample time. Initial conditions are sampled automatically.
      mask Display: fprintf('%.2f Hz lowpass',f)
  Add : Sum  Inputs=+-  OutScaling=2^-10  SampleTime=apSampleTime
  Add1 : Sum  Inputs=3  OutDataTypeMode=single  OutScaling=2^-10  SampleTime=apSampleTime
  Add2 : Sum  Inputs=+-  OutDataTypeMode=single  OutScaling=2^-10  SampleTime=apSampleTime
  Add3 : Sum  Inputs=+-  OutDataTypeMode=single  OutScaling=2^-10
  Add4 : Sum  Inputs=3  OutDataTypeMode=single  OutScaling=2^-10
  Add5 : Sum  Inputs=+-  OutDataTypeMode=single  OutScaling=2^-10
  Air Density from Height : Subsystem
  Airspeed Hold [PID] : Subsystem  AncestorBlock=SLUGS_Library/Control Blocks/PID Controller w//Anti-Windup  mask(PID){Tsample=apSampleTime, Ndelay=derivativesConstant, upperSaturationLimit=dtLimit, lowerSaturationLimit=0}
      mask prompts: Tsample "Sample Time"; Ndelay "Integer delays for de/dt"; upperSaturationLimit "Upper Saturation Limit"; lowerSaturationLimit "Lower Saturation Limit"
      mask help: PID controller block with anti-windup and saturation limits. Implemented as a discrete forwardl integration which stops integrating when the output is saturated. Derivative is implemented as a numerical derivative with N integer delays to smooth output.
      mask Display:
      | disp('PID')
      | port_label('input',1,'error')
      | port_label('input',3,'gains')
      | port_label('input',2,'reset')
      | port_label('input',4,'trim')
      | port_label('output',1,'output')
  Compute Airspeed : Subsystem
  Constant1 : Constant  Value=0  OutDataTypeMode=single
  Constant2 : Constant  OutDataTypeMode=single
  Constant4 : Constant  OutDataTypeMode=single
  Elevator  Limit : Saturate  UpperLimit=deLimit  LowerLimit=-deLimit  SampleTime=apSampleTime
  Height Error to Pitch  Command [PI] : SLUGS_Library/Control Blocks/PI Controller w//Anti-Windup  SystemSampleTime=-1  Tsample=apSampleTime  Ndelay=derivativesConstant  upperSaturationLimit=pitchCommandLimit  lowerSaturationLimit=-pitchCommandLimit
  Manual?1 : InportShadow  Port=11  LatchByCopyingInsideSignal=off
  Manual?2 : InportShadow  Port=11  LatchByCopyingInsideSignal=off
  Pitch To Elevator [PID] : SLUGS_Library/Control Blocks/PID Controller w//Anti-Windup  SystemSampleTime=-1  Tsample=apSampleTime  Ndelay=derivativesConstant  upperSaturationLimit=deLimit  lowerSaturationLimit=-deLimit
  Product : Product  Inputs=*/  RndMeth=Zero
  Product1 : Product  RndMeth=Zero
  Product2 : Product  RndMeth=Zero
  Rate Limiter : RateLimiter  RisingSlewLimit=7  FallingSlewLimit=-5  SampleTimeMode=inherited  InitialCondition=Pos_0(3)
  Schedule LPF : Switch  Criteria=u2 > Threshold  Threshold=0.3
  Subsystem5 : Subsystem  AncestorBlock=SLUGS_Library/Subsystem5
  Switch : Switch  Criteria=u2 > Threshold  Threshold=0.3  SampleTime=apSampleTime  InputSameDT=on
  Theta_c Limit : Saturate  UpperLimit=pitchCommandLimit  LowerLimit=-8*pi/180  SampleTime=apSampleTime
  Throttle  Limit : Saturate  UpperLimit=dtLimit  LowerLimit=0  SampleTime=apSampleTime
  Use D Term for FF Must be Negative : Selector  IndexOptions=Index vector (dialog)  Indices=3  OutputSizes=1  InputPortWidth=3
  "[-60 60]" : Saturate  UpperLimit=60  LowerLimit=-60  SampleTime=apSampleTime
  h_m1 : InportShadow  Port=6  LatchByCopyingInsideSignal=off
  lowpass limit : simulink/Logic and Bit Operations/Compare To Constant  SystemSampleTime=-1  relop=<=  const=10.0  LogicOutDataTypeMode=uint8  ZeroCross=off
  "theta_m " : InportShadow  Port=8  LatchByCopyingInsideSignal=off
  dE : Outport
  dT : Outport  Port=2
  theta_C : Outport  Port=3
  h_c_in : Outport  Port=4
  U_m : Outport  Orientation=left  Port=5
  wires:
  U_c/1 -> Add/1
  Add/1 -> Airspeed Hold [PID]/1(Error)
  Airspeed Hold [PID]/1(Output) -> Add1/1
  dT_trim/1 -> Add1/2, Airspeed Hold [PID]/4(Trim)
  Add1/1 -> Throttle  Limit/1
  Throttle  Limit/1 -> dT/1
  Add2/1 -> Height Error to Pitch  Command [PI]/1
  h_m/1 -> Add2/2
  theta_m/1 -> Add3/2
  Manual?/1 -> Airspeed Hold [PID]/2(Reset)
  Manual?1/1 -> Height Error to Pitch  Command [PI]/2
  Manual?2/1 -> Pitch To Elevator [PID]/2
  Add4/1 -> Elevator  Limit/1
  Pitch To Elevator [PID]/1 -> Add4/1
  dE_trim/1 -> Add4/2, Pitch To Elevator [PID]/4
  Elevator  Limit/1 -> dE/1
  Air Density from Height/1(rho (Kg/m^3)) -> Compute Airspeed/2(rho)
  dyn P/1 -> Compute Airspeed/1(Dyn P)
  h_m1/1 -> Air Density from Height/1(h(m))
  Add3/1 -> Pitch To Elevator [PID]/1
  Theta_c Limit/1 -> Add3/1, theta_C/1
  wpFly/1 -> Switch/2
  Switch/1 -> Rate Limiter/1
  h_c/1 -> Switch/3
  h__nav_c/1 -> Switch/1
  Rate Limiter/1 -> Add2/1, h_c_in/1
  Height Error to Pitch  Command [PI]/1 -> Theta_c Limit/1
  Constant2/1 -> Add5/2
  Subsystem5/1(cos(u)) -> Product/2
  Constant4/1 -> Product/1
  Product/1 -> Add5/1
  0.5 sec  tau for Turns/1(Out1) -> "[-60 60]"/1
  "[-60 60]"/1 -> Subsystem5/1(u)
  phi_m/1 -> 0.5 sec  tau for Turns/1(In1)
  Use D Term for FF Must be Negative/1 -> Product1/1
  Product1/1 -> Add4/3
  Add5/1 -> Product1/2
  Compute Airspeed/1(Airspeed m(s)) -> 0.3 sec  tau for low speeds/1(In1), 5 sec tau for high speeds/1(In1), lowpass limit/1
  Schedule LPF/1 -> Add/2, U_m/1
  U_hold PID Gains/1 -> Airspeed Hold [PID]/3(PIDGains)
  "theta_m "/1 -> Product2/2
  dt FF Gain/1 -> Product2/1
  Product2/1 -> Add1/3
  lowpass limit/1 -> Schedule LPF/2
  5 sec tau for high speeds/1(Out1) -> Schedule LPF/3
  0.3 sec  tau for low speeds/1(Out1) -> Schedule LPF/1
  he2th PID Gains/1 -> Height Error to Pitch  Command [PI]/3, Use D Term for FF Must be Negative/1
  Constant1/1 -> Height Error to Pitch  Command [PI]/4
  th2dE PID Gains/1 -> Pitch To Elevator [PID]/3

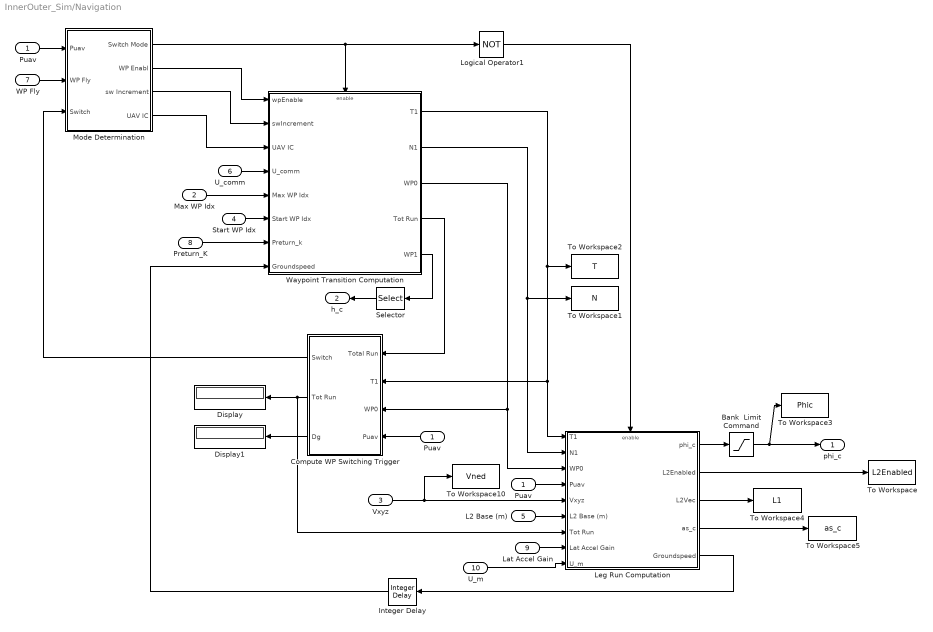
== system InnerOuter_Sim/Navigation ==
  Puav : Inport  SampleTime=apSampleTime
  Max WP Idx : Inport  Port=2
  Vxyz : Inport  Port=3
  Start WP Idx : Inport  Port=4
  L2 Base (m) : Inport  Port=5
  U_comm : Inport  Port=6
  WP Fly : Inport  Port=7
  Preturn_K : Inport  Port=8
  Lat Accel Gain : Inport  Port=9
  U_m : Inport  Port=10
  Bank  Limit Command : Saturate  UpperLimit=bankCommandLimit  LowerLimit=-bankCommandLimit  SampleTime=apSampleTime
  Compute WP Switching Trigger : Subsystem  Orientation=left
  Display : Display
  Display1 : Display
  Integer Delay : simulink/Discrete/Integer Delay  Orientation=left  vinit=0.0  samptime=-1  NumDelays=1
  Leg Run Computation : Subsystem
  Logical Operator1 : Logic  Operator=NOT  AllPortsSameDT=off  OutDataTypeMode=Boolean
  Mode Determination : Subsystem
  "Puav " : InportShadow  Port=1  SampleTime=apSampleTime  LatchByCopyingInsideSignal=off
  "Puav  " : InportShadow  Orientation=left  Port=1  SampleTime=apSampleTime  LatchByCopyingInsideSignal=off
  Selector : Selector  Orientation=left  IndexOptions=Index vector (dialog)  Indices=[3]  OutputSizes=1  InputPortWidth=3
  To Workspace : ToWorkspace  VariableName=L2Enabled  SampleTime=-1  SaveFormat=Array
  To Workspace1 : ToWorkspace  VariableName=N  SampleTime=-1  SaveFormat=Array
  To Workspace10 : ToWorkspace  VariableName=Vned  SampleTime=-1  SaveFormat=Array
  To Workspace2 : ToWorkspace  VariableName=T  SampleTime=-1  SaveFormat=Array
  To Workspace3 : ToWorkspace  VariableName=Phic  SampleTime=-1  SaveFormat=Array
  To Workspace4 : ToWorkspace  VariableName=L1  SampleTime=-1  SaveFormat=Array
  To Workspace5 : ToWorkspace  VariableName=as_c  SampleTime=-1  SaveFormat=Array
  Waypoint Transition Computation : Subsystem
  phi_c : Outport
  h_c : Outport  Orientation=left  Port=2
  wires:
  Mode Determination/2(WP Enabl) -> Waypoint Transition Computation/1(wpEnable)
  Mode Determination/3(sw Increment) -> Waypoint Transition Computation/2(swIncrement)
  U_comm/1 -> Waypoint Transition Computation/4(U_comm)
  Max WP Idx/1 -> Waypoint Transition Computation/5(Max WP Idx)
  Start WP Idx/1 -> Waypoint Transition Computation/6(Start WP Idx)
  Mode Determination/1(Switch Mode) -> Waypoint Transition Computation/Enable, Logical Operator1/1
  Logical Operator1/1 -> Leg Run Computation/Enable
  L2 Base (m)/1 -> Leg Run Computation/6(L2 Base (m))
  Vxyz/1 -> Leg Run Computation/5(Vxyz), To Workspace10/1
  "Puav "/1 -> Leg Run Computation/4(Puav)
  Waypoint Transition Computation/1(T1) -> Leg Run Computation/1(T1), Compute WP Switching Trigger/2(T1), To Workspace2/1
  Waypoint Transition Computation/2(N1) -> Leg Run Computation/2(N1), To Workspace1/1
  Waypoint Transition Computation/3(WP0) -> Leg Run Computation/3(WP0), Compute WP Switching Trigger/3(WP0)
  "Puav  "/1 -> Compute WP Switching Trigger/4(Puav)
  Waypoint Transition Computation/4(Tot Run) -> Compute WP Switching Trigger/1(Total Run)
  Selector/1 -> h_c/1
  Waypoint Transition Computation/5(WP1) -> Selector/1
  Mode Determination/4(UAV IC) -> Waypoint Transition Computation/3(UAV IC)
  Puav/1 -> Mode Determination/1(Puav)
  WP Fly/1 -> Mode Determination/2(WP Fly)
  Compute WP Switching Trigger/1(Switch) -> Mode Determination/3(Switch)
  Compute WP Switching Trigger/2(Tot Run) -> Display/1, Leg Run Computation/7(Tot Run)
  Compute WP Switching Trigger/3(Dg) -> Display1/1
  Leg Run Computation/2(L2Enabled) -> To Workspace/1
  Leg Run Computation/3(L2Vec) -> To Workspace4/1
  Leg Run Computation/1(phi_c) -> Bank  Limit Command/1
  Leg Run Computation/4(as_c) -> To Workspace5/1
  Bank  Limit Command/1 -> phi_c/1, To Workspace3/1
  Preturn_K/1 -> Waypoint Transition Computation/7(Preturn_k)
  Leg Run Computation/5(Groundspeed) -> Integer Delay/1
  Integer Delay/1 -> Waypoint Transition Computation/8(Groundspeed)
  Lat Accel Gain/1 -> Leg Run Computation/8(Lat Accel Gain)
  U_m/1 -> Leg Run Computation/9(U_m)

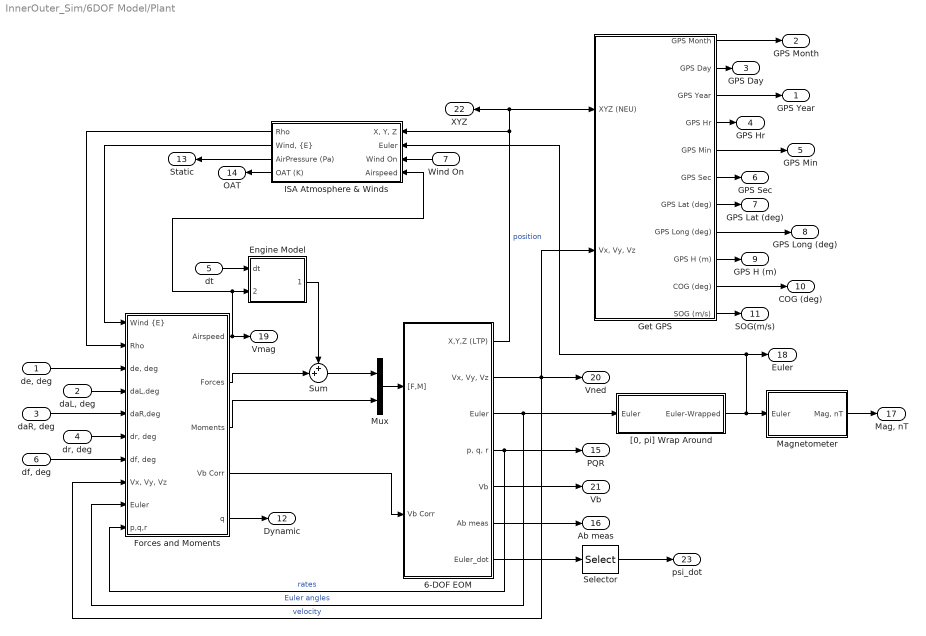
== system InnerOuter_Sim/6DOF Model/Plant ==
  "de, deg" : Inport
  "daL, deg" : Inport  Port=2
  "daR, deg" : Inport  Port=3
  "dr, deg" : Inport  Port=4
  dt : Inport  Port=5
  "df, deg" : Inport  Port=6
  Wind On : Inport  Orientation=left  Port=7
  6-DOF EOM : Subsystem
  Engine Model : Subsystem
  Forces and Moments : Subsystem
  Get GPS : Subsystem
  ISA Atmosphere & Winds : Subsystem  Orientation=left
  Magnetometer : Subsystem  mask{magField=[ 23143.6 5858.2 45511.9]}
      mask prompts: magField "Local Magnetic Field"
      mask help:
      | Simulates the Data from magnetometers with no noise.
      |
      | You can obtain data for the local magnetic field at:
      |
      | http://www.ngdc.noaa.gov/geomagmodels/IGRFWMM.jsp
  Mux : Mux  Inputs=2
  Selector : Selector  IndexOptions=Index vector (dialog)  Indices=[3]  OutputSizes=1  InputPortWidth=3
  Sum : Sum  Inputs=++|  SaturateOnIntegerOverflow=on
  "[0, pi] Wrap Around" : Subsystem
  GPS Year : Outport
  GPS Month : Outport  Port=2
  GPS Day : Outport  Port=3
  GPS Hr : Outport  Port=4
  GPS Min : Outport  Port=5
  GPS Sec : Outport  Port=6
  GPS Lat (deg) : Outport  Port=7
  GPS Long (deg) : Outport  Port=8
  GPS H (m) : Outport  Port=9
  COG (deg) : Outport  Port=10
  SOG(m/s) : Outport  Port=11
  Dynamic : Outport  Port=12
  Static : Outport  Orientation=left  Port=13
  OAT : Outport  Orientation=left  Port=14
  PQR : Outport  Port=15
  Ab meas : Outport  Port=16
  "Mag, nT" : Outport  Port=17
  Euler : Outport  Port=18
  Vmag : Outport  Port=19
  Vned : Outport  Port=20
  Vb : Outport  Port=21
  XYZ : Outport  Orientation=left  Port=22
  psi_dot : Outport  Port=23
  wires:
  Get GPS/1(GPS Month) -> GPS Month/1
  Get GPS/2(GPS Day) -> GPS Day/1
  Get GPS/3(GPS Year) -> GPS Year/1
  Get GPS/4(GPS Hr) -> GPS Hr/1
  Get GPS/5(GPS Min) -> GPS Min/1
  Get GPS/6(GPS Sec) -> GPS Sec/1
  Get GPS/7(GPS Lat (deg)) -> GPS Lat (deg)/1
  Get GPS/8(GPS Long (deg)) -> GPS Long (deg)/1
  Get GPS/9(GPS H (m)) -> GPS H (m)/1
  6-DOF EOM/6(Ab meas) -> Ab meas/1
  Mux/1 -> 6-DOF EOM/1("[F,M]")
  6-DOF EOM/5(Vb) -> Vb/1
  Engine Model/1(Thrust) -> Sum/1
  Forces and Moments/5(q) -> Dynamic/1
  ISA Atmosphere & Winds/3(AirPressure (Pa)) -> Static/1
  Forces and Moments/1(Airspeed) -> Vmag/1, Engine Model/2(Vmag), ISA Atmosphere & Winds/4(Airspeed)
  ISA Atmosphere & Winds/2("Wind, {E}") -> Forces and Moments/1("Wind {E}")
  ISA Atmosphere & Winds/1(Rho) -> Forces and Moments/2(Rho)
  Forces and Moments/3(Moments) -> Mux/2
  Forces and Moments/2(Forces) -> Sum/2
  Sum/1 -> Mux/1
  Forces and Moments/4(Vb Corr) -> 6-DOF EOM/2(Vb Corr)
  6-DOF EOM/1(X,Y,Z (LTP)) -> ISA Atmosphere & Winds/1("X, Y, Z"), Get GPS/1(XYZ (NEU)), XYZ/1  "position"
  6-DOF EOM/2("Vx, Vy, Vz") -> Vned/1, Get GPS/2("Vx, Vy, Vz"), Forces and Moments/8("Vx, Vy, Vz ")  "velocity"
  6-DOF EOM/3(Euler) -> "[0, pi] Wrap Around"/1(Euler), Forces and Moments/9(Euler)  "Euler angles"
  6-DOF EOM/4("p, q, r") -> PQR/1, Forces and Moments/10(p,q,r)  "rates"
  dt/1 -> Engine Model/1(dt)
  "de, deg"/1 -> Forces and Moments/3("de, deg")
  "daL, deg"/1 -> Forces and Moments/4(daL,deg)
  "dr, deg"/1 -> Forces and Moments/6("dr, deg")
  "df, deg"/1 -> Forces and Moments/7("df, deg")
  "[0, pi] Wrap Around"/1(Euler-Wrapped) -> Magnetometer/1(Euler), Euler/1, ISA Atmosphere & Winds/2(Euler)
  Magnetometer/1("Mag, nT") -> "Mag, nT"/1
  Get GPS/10(COG (deg)) -> COG (deg)/1
  Get GPS/11(SOG (m/s)) -> SOG(m/s)/1
  ISA Atmosphere & Winds/4(OAT (K)) -> OAT/1
  6-DOF EOM/7(Euler_dot) -> Selector/1
  Selector/1 -> psi_dot/1
  Wind On/1 -> ISA Atmosphere & Winds/3(Wind On)
  "daR, deg"/1 -> Forces and Moments/5(daR,deg)
